simulink model "bh_SM_quad_NO_spin_props"  (R2017a)
settings: Solver=ode23t  StartTime=0.0  StopTime=200  FixedStep=0.001  RelTol=1e-5  EnableMultiTasking=on
undefined symbols (not defined in the file): P_elec, P_mot, P_one_prop, P_rot, P_veh, P_veh_no_props, sigbuilder_block, X, xme_dot_0, Y, Z
libraries: bh_6dof_LIBRARY x22, sm_lib x22, nesl_utility x19, simulink_extras x17, simulink x15
(part 2 of 3)

== system bh_SM_quad_NO_spin_props/CONT_SYS Force_Moment_CMDS/PITCH_and_ROLL_CONT/plots ==
  In1 : Inport
  Demux : Demux  Outputs=2
  Demux1 : Demux  Outputs=2
  P_and_R_CMDs : Scope  NumInputPorts=6
  Radians to Degrees : simulink_extras/Transformations/Radians to Degrees
  Radians to Degrees1 : simulink_extras/Transformations/Radians to Degrees
  Radians to Degrees2 : simulink_extras/Transformations/Radians to Degrees
  wires:
  In1/1 -> Demux1/1, Radians to Degrees/1, Demux/1, P_and_R_CMDs/1
  Demux/1 -> P_and_R_CMDs/2  "Pitch_rad"
  Demux/2 -> P_and_R_CMDs/3  "Roll_rad"
  Radians to Degrees/1 -> P_and_R_CMDs/4  "p_and_r_DEG"
  Demux1/1 -> Radians to Degrees2/1
  Demux1/2 -> Radians to Degrees1/1
  Radians to Degrees2/1 -> P_and_R_CMDs/5  "Pitch_DEG"
  Radians to Degrees1/1 -> P_and_R_CMDs/6  "Roll_DEG"

== system bh_SM_quad_NO_spin_props/CONT_SYS Force_Moment_CMDS/PITCH_and_ROLL_CONT/psi ==
  In1 : Inport
  Bus Selector1 : BusSelector  OutputSignals=phi_theta_psi
  Bus Selector2 : BusSelector  OutputSignals=DOT_phi_theta_psi
  Selector1 : Selector  InputPortWidth=3  IndexOptions=Index vector (dialog)  Indices=3  OutputSizes=1
  Selector2 : Selector  InputPortWidth=3  IndexOptions=Index vector (dialog)  Indices=3  OutputSizes=1
  Out1 : Outport
  Out2 : Outport  Port=2
  wires:
  In1/1 -> Bus Selector2/1, Bus Selector1/1
  Selector1/1 -> Out1/1
  Bus Selector1/1 -> Selector1/1  "<phi_theta_psi>"
  Bus Selector2/1 -> Selector2/1  "<DOT_phi_theta_psi>"
  Selector2/1 -> Out2/1

== system bh_SM_quad_NO_spin_props/CONT_SYS Force_Moment_CMDS/PITCH_and_ROLL_CONT/theta ==
  In1 : Inport
  Bus Selector1 : BusSelector  OutputSignals=phi_theta_psi
  Bus Selector2 : BusSelector  OutputSignals=DOT_phi_theta_psi
  Selector1 : Selector  InputPortWidth=3  IndexOptions=Index vector (dialog)  Indices=2  OutputSizes=1
  Selector2 : Selector  InputPortWidth=3  IndexOptions=Index vector (dialog)  Indices=2  OutputSizes=1
  Out1 : Outport
  Out2 : Outport  Port=2
  wires:
  In1/1 -> Bus Selector2/1, Bus Selector1/1
  Selector1/1 -> Out1/1
  Bus Selector1/1 -> Selector1/1  "<phi_theta_psi>"
  Bus Selector2/1 -> Selector2/1  "<DOT_phi_theta_psi>"
  Selector2/1 -> Out2/1

== system bh_SM_quad_NO_spin_props/CONT_SYS Force_Moment_CMDS/YAW_CONT/FINAL_DES_YAW_CONTROL_SYSTEM ==
  note: NOTE: 1 radian = 57 degrees
  YAW_CMD : Inport
  YAW_MEAS : Inport  Port=2
  YAW_dot_MEAS : Inport  Port=3
  P_CONT_too : simulink/Continuous/PID Controller  Controller=P  TimeDomain=Continuous-time  SampleTime=-1  IntegratorMethod=Forward Euler  FilterMethod=Forward Euler  Form=Parallel  UseFilter=on  ControllerParametersSource=internal  P=1.61636567778084  I=0.151389824684851  D=0  N=100  InitialConditionSource=internal  InitialConditionForIntegrator=0  InitialConditionForFilter=0  ExternalReset=none  LimitOutput=off  UpperSaturationLimit=inf  LowerSaturationLimit=-inf  LinearizeAsGain=on  AntiWindupMode=none  Kb=1  TrackingMode=off  Kt=1  PParamMin=[]  PParamMax=[]  IParamMin=[]  IParamMax=[]  DParamMin=[]  DParamMax=[]  NParamMin=[]  NParamMax=[]  KbParamMin=[]  KbParamMax=[]  KtParamMin=[]  KtParamMax=[]  POutMin=[]  POutMax=[]  IOutMin=[]  IOutMax=[]  DOutMin=[]  DOutMax=[]  NOutMin=[]  NOutMax=[]  KbOutMin=[]  KbOutMax=[]  KtOutMin=[]  KtOutMax=[]  IntegratorOutMin=[]  IntegratorOutMax=[]  FilterOutMin=[]  FilterOutMax=[]  SumOutMin=[]  SumOutMax=[]  SumI1OutMin=[]  SumI1OutMax=[]  SumI2OutMin=[]  SumI2OutMax=[]  SumI3OutMin=[]  SumI3OutMax=[]  SumDOutMin=[]  SumDOutMax=[]  SaturationOutMin=[]  SaturationOutMax=[]  IntegratorContinuousStateAttributes=''  IntegratorStateMustResolveToSignalObject=off  IntegratorRTWStateStorageClass=Auto  FilterContinuousStateAttributes=''  FilterStateMustResolveToSignalObject=off  FilterRTWStateStorageClass=Auto  DifferentiatorICPrevScaledInput=0  DifferentiatorOutMin=[]  DifferentiatorOutMax=[]  InitialConditionSetting=State (most efficient)
  P_Cont : simulink/Continuous/PID Controller  Controller=P  TimeDomain=Continuous-time  SampleTime=-1  IntegratorMethod=Forward Euler  FilterMethod=Forward Euler  Form=Parallel  UseFilter=on  ControllerParametersSource=internal  P=0.09744859506471  I=7.09690484808648  D=-0.334898279224841  N=17.076664592689  InitialConditionSource=internal  InitialConditionForIntegrator=0  InitialConditionForFilter=0  ExternalReset=none  LimitOutput=off  UpperSaturationLimit=inf  LowerSaturationLimit=-inf  LinearizeAsGain=on  AntiWindupMode=none  Kb=1  TrackingMode=off  Kt=1  PParamMin=[]  PParamMax=[]  IParamMin=[]  IParamMax=[]  DParamMin=[]  DParamMax=[]  NParamMin=[]  NParamMax=[]  KbParamMin=[]  KbParamMax=[]  KtParamMin=[]  KtParamMax=[]  POutMin=[]  POutMax=[]  IOutMin=[]  IOutMax=[]  DOutMin=[]  DOutMax=[]  NOutMin=[]  NOutMax=[]  KbOutMin=[]  KbOutMax=[]  KtOutMin=[]  KtOutMax=[]  IntegratorOutMin=[]  IntegratorOutMax=[]  FilterOutMin=[]  FilterOutMax=[]  SumOutMin=[]  SumOutMax=[]  SumI1OutMin=[]  SumI1OutMax=[]  SumI2OutMin=[]  SumI2OutMax=[]  SumI3OutMin=[]  SumI3OutMax=[]  SumDOutMin=[]  SumDOutMax=[]  SaturationOutMin=[]  SaturationOutMax=[]  IntegratorContinuousStateAttributes=''  IntegratorStateMustResolveToSignalObject=off  IntegratorRTWStateStorageClass=Auto  FilterContinuousStateAttributes=''  FilterStateMustResolveToSignalObject=off  FilterRTWStateStorageClass=Auto  DifferentiatorICPrevScaledInput=0  DifferentiatorOutMin=[]  DifferentiatorOutMax=[]  InitialConditionSetting=State (most efficient)
  Sum1 : Sum  Inputs=|+-
  Sum3 : Sum  Inputs=|+-
  TQ_YAW : Outport
  wires:
  Sum3/1 -> P_Cont/1
  P_Cont/1 -> TQ_YAW/1  "TQ"
  YAW_CMD/1 -> Sum1/1
  YAW_MEAS/1 -> Sum1/2
  YAW_dot_MEAS/1 -> Sum3/2
  Sum1/1 -> P_CONT_too/1
  P_CONT_too/1 -> Sum3/1

== system bh_SM_quad_NO_spin_props/CONT_SYS Force_Moment_CMDS/Z_CONT/FINAL_DES_ALTITUDE_CONTROL_SYSTEM ==
  Ze_CMD : Inport
  Ze_MEAS : Inport  Port=2
  Ze_dot_MEAS : Inport  Port=3
  P_cont : simulink/Continuous/PID Controller  Controller=P  TimeDomain=Continuous-time  SampleTime=-1  IntegratorMethod=Forward Euler  FilterMethod=Forward Euler  Form=Parallel  UseFilter=on  ControllerParametersSource=internal  P=6.7862699178667  I=7.09690484808648  D=-0.334898279224841  N=17.076664592689  InitialConditionSource=internal  InitialConditionForIntegrator=0  InitialConditionForFilter=0  ExternalReset=none  LimitOutput=off  UpperSaturationLimit=inf  LowerSaturationLimit=-inf  LinearizeAsGain=on  AntiWindupMode=none  Kb=1  TrackingMode=off  Kt=1  PParamMin=[]  PParamMax=[]  IParamMin=[]  IParamMax=[]  DParamMin=[]  DParamMax=[]  NParamMin=[]  NParamMax=[]  KbParamMin=[]  KbParamMax=[]  KtParamMin=[]  KtParamMax=[]  POutMin=[]  POutMax=[]  IOutMin=[]  IOutMax=[]  DOutMin=[]  DOutMax=[]  NOutMin=[]  NOutMax=[]  KbOutMin=[]  KbOutMax=[]  KtOutMin=[]  KtOutMax=[]  IntegratorOutMin=[]  IntegratorOutMax=[]  FilterOutMin=[]  FilterOutMax=[]  SumOutMin=[]  SumOutMax=[]  SumI1OutMin=[]  SumI1OutMax=[]  SumI2OutMin=[]  SumI2OutMax=[]  SumI3OutMin=[]  SumI3OutMax=[]  SumDOutMin=[]  SumDOutMax=[]  SaturationOutMin=[]  SaturationOutMax=[]  IntegratorContinuousStateAttributes=''  IntegratorStateMustResolveToSignalObject=off  IntegratorRTWStateStorageClass=Auto  FilterContinuousStateAttributes=''  FilterStateMustResolveToSignalObject=off  FilterRTWStateStorageClass=Auto  DifferentiatorICPrevScaledInput=0  DifferentiatorOutMin=[]  DifferentiatorOutMax=[]  InitialConditionSetting=State (most efficient)
  P_cont_too : simulink/Continuous/PID Controller  Controller=P  TimeDomain=Continuous-time  SampleTime=-1  IntegratorMethod=Forward Euler  FilterMethod=Forward Euler  Form=Parallel  UseFilter=on  ControllerParametersSource=internal  P=0.931782439164433  I=0.151389824684851  D=0.117353405685993  N=2.94633103429336  InitialConditionSource=internal  InitialConditionForIntegrator=0  InitialConditionForFilter=0  ExternalReset=none  LimitOutput=off  UpperSaturationLimit=inf  LowerSaturationLimit=-inf  LinearizeAsGain=on  AntiWindupMode=none  Kb=1  TrackingMode=off  Kt=1  PParamMin=[]  PParamMax=[]  IParamMin=[]  IParamMax=[]  DParamMin=[]  DParamMax=[]  NParamMin=[]  NParamMax=[]  KbParamMin=[]  KbParamMax=[]  KtParamMin=[]  KtParamMax=[]  POutMin=[]  POutMax=[]  IOutMin=[]  IOutMax=[]  DOutMin=[]  DOutMax=[]  NOutMin=[]  NOutMax=[]  KbOutMin=[]  KbOutMax=[]  KtOutMin=[]  KtOutMax=[]  IntegratorOutMin=[]  IntegratorOutMax=[]  FilterOutMin=[]  FilterOutMax=[]  SumOutMin=[]  SumOutMax=[]  SumI1OutMin=[]  SumI1OutMax=[]  SumI2OutMin=[]  SumI2OutMax=[]  SumI3OutMin=[]  SumI3OutMax=[]  SumDOutMin=[]  SumDOutMax=[]  SaturationOutMin=[]  SaturationOutMax=[]  IntegratorContinuousStateAttributes=''  IntegratorStateMustResolveToSignalObject=off  IntegratorRTWStateStorageClass=Auto  FilterContinuousStateAttributes=''  FilterStateMustResolveToSignalObject=off  FilterRTWStateStorageClass=Auto  DifferentiatorICPrevScaledInput=0  DifferentiatorOutMin=[]  DifferentiatorOutMax=[]  InitialConditionSetting=State (most efficient)
  Sum1 : Sum  Inputs=|+-
  Sum3 : Sum  Inputs=|+-
  THRUST : Outport
  wires:
  Sum1/1 -> P_cont_too/1
  Sum3/1 -> P_cont/1
  Ze_CMD/1 -> Sum1/1
  P_cont/1 -> THRUST/1  "THRUST"
  P_cont_too/1 -> Sum3/1
  Ze_MEAS/1 -> Sum1/2
  Ze_dot_MEAS/1 -> Sum3/2

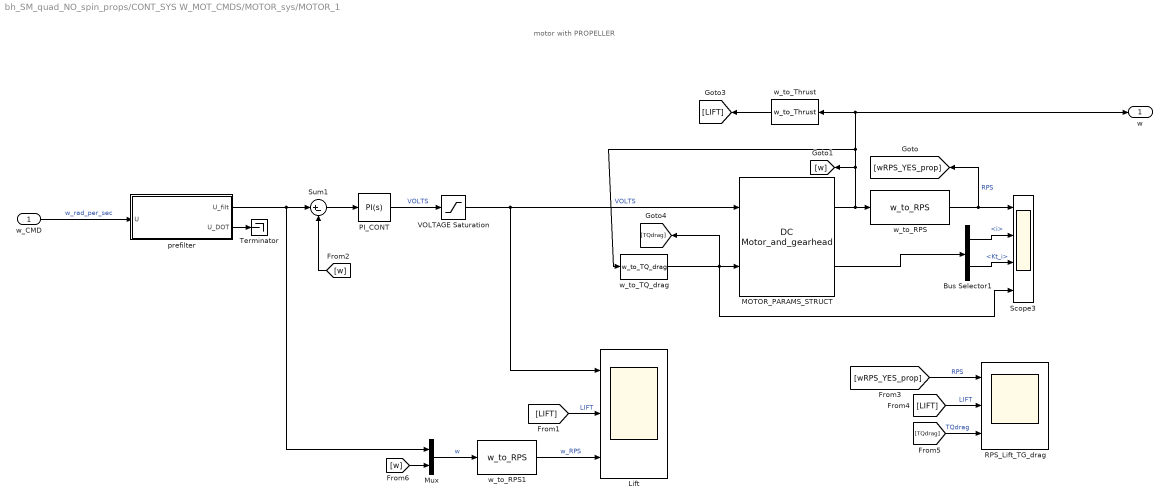
== system bh_SM_quad_NO_spin_props/CONT_SYS W_MOT_CMDS/MOTOR_sys/MOTOR_1 ==
  note: motor with PROPELLER
  w_CMD : Inport
  Bus Selector1 : BusSelector  OutputSignals=Elec.i,TQ_mot.Kt_i
  Lift : Scope  NumInputPorts=3
  MOTOR_PARAMS_STRUCT : bh_6dof_LIBRARY/MODELS/DC Motor_and_gearhead  K=P_mot.Ka  B=P_mot.b  J=P_mot.I  R=P_mot.R  L=P_mot.L  Kb=P_mot.Ke  ID=P_mot.ID
  Mux : Mux  Inputs=2
  PI_CONT : simulink/Continuous/PID Controller  Controller=PI  TimeDomain=Continuous-time  SampleTime=-1  IntegratorMethod=Forward Euler  FilterMethod=Forward Euler  Form=Parallel  UseFilter=on  ControllerParametersSource=internal  P=2.97678216835849  I=24.9655384194189  D=-0.0417302954853434  N=6.67624174583517  InitialConditionSource=internal  InitialConditionForIntegrator=0  InitialConditionForFilter=0  ExternalReset=none  LimitOutput=off  UpperSaturationLimit=inf  LowerSaturationLimit=-inf  LinearizeAsGain=on  AntiWindupMode=none  Kb=1  TrackingMode=off  Kt=1  PParamMin=[]  PParamMax=[]  IParamMin=[]  IParamMax=[]  DParamMin=[]  DParamMax=[]  NParamMin=[]  NParamMax=[]  KbParamMin=[]  KbParamMax=[]  KtParamMin=[]  KtParamMax=[]  POutMin=[]  POutMax=[]  IOutMin=[]  IOutMax=[]  DOutMin=[]  DOutMax=[]  NOutMin=[]  NOutMax=[]  KbOutMin=[]  KbOutMax=[]  KtOutMin=[]  KtOutMax=[]  IntegratorOutMin=[]  IntegratorOutMax=[]  FilterOutMin=[]  FilterOutMax=[]  SumOutMin=[]  SumOutMax=[]  SumI1OutMin=[]  SumI1OutMax=[]  SumI2OutMin=[]  SumI2OutMax=[]  SumI3OutMin=[]  SumI3OutMax=[]  SumDOutMin=[]  SumDOutMax=[]  SaturationOutMin=[]  SaturationOutMax=[]  IntegratorContinuousStateAttributes=''  IntegratorStateMustResolveToSignalObject=off  IntegratorRTWStateStorageClass=Auto  FilterContinuousStateAttributes=''  FilterStateMustResolveToSignalObject=off  FilterRTWStateStorageClass=Auto  DifferentiatorICPrevScaledInput=0  DifferentiatorOutMin=[]  DifferentiatorOutMax=[]  InitialConditionSetting=State (most efficient)
  RPS_Lift_TG_drag : Scope  NumInputPorts=3
  Scope3 : Scope  NumInputPorts=4
  Sum1 : Sum  Inputs=|+-
  Terminator : Terminator
  VOLTAGE Saturation : Saturate  UpperLimit=P_elec.V_mot_max  LowerLimit=P_elec.V_mot_min
      settings: AttributesFormatString=|
      | Vmax = %<UpperLimit>
      | Vmin = %<LowerLimit>
  prefilter : Subsystem  mask(Derivative Estimation){wn=2*pi*5, p=1}
      mask prompts: wn "Natural frequency, wn (rad/sec)"; p "Damping ratio, p"
      mask help:
      | A simple derivative estimator using a 2nd order representation between input and output.
      |
      | The integrators use a discrete FORWARd Euler rule, and a sample time needs to be specified.
      mask init:
      | str1 = sprintf('wn = %.2f', wn);
      | str2 = sprintf('p  = %.2f', p);
      | %str3 = sprintf('dt = %.2f', dt);
      | %str = char(str1,str2,str3);
      | %str3 = sprintf('dt = %.2f', dt);
      | str = char(str1,str2);
      mask Display: disp(str)
  w_to_RPS : bh_6dof_LIBRARY/MODELS/w_to_RPS  SystemSampleTime=-1
  w_to_RPS1 : bh_6dof_LIBRARY/MODELS/w_to_RPS  SystemSampleTime=-1
  w_to_TQ_drag : bh_6dof_LIBRARY/MODELS/w_to_TQ_drag  k=P_one_prop.TWIST_per_w2
  w_to_Thrust : bh_6dof_LIBRARY/MODELS/w_to_Thrust  k=P_one_prop.LIFT_per_w2
  w : Outport
  wires:
  VOLTAGE Saturation/1 -> Lift/1, MOTOR_PARAMS_STRUCT/1  "VOLTS"
  [TQdrag] -> RPS_Lift_TG_drag/3  "TQdrag"
  Sum1/1 -> PI_CONT/1
  w_to_TQ_drag/1 -> [TQdrag], MOTOR_PARAMS_STRUCT/2, Scope3/4
  [LIFT] -> RPS_Lift_TG_drag/2  "LIFT"
  [wRPS_YES_prop] -> RPS_Lift_TG_drag/1  "RPS"
  w_to_Thrust/1 -> [LIFT]
  w_to_RPS/1 -> [wRPS_YES_prop], Scope3/1  "RPS"
  Bus Selector1/1 -> Scope3/2  "<i>"
  MOTOR_PARAMS_STRUCT/2 -> Bus Selector1/1
  Bus Selector1/2 -> Scope3/3  "<Kt_i>"
  MOTOR_PARAMS_STRUCT/1 -> w_to_RPS/1, [w], w/1, w_to_Thrust/1, w_to_TQ_drag/1
  [w] -> Sum1/2
  [LIFT] -> Lift/2  "LIFT"
  Mux/1 -> w_to_RPS1/1  "w"
  [w] -> Mux/2
  w_to_RPS1/1 -> Lift/3  "w_RPS"
  PI_CONT/1 -> VOLTAGE Saturation/1  "VOLTS"
  w_CMD/1 -> prefilter/1(U)  "w_rad_per_sec"
  prefilter/1(U_filt) -> Mux/1, Sum1/1
  prefilter/2(U_DOT) -> Terminator/1

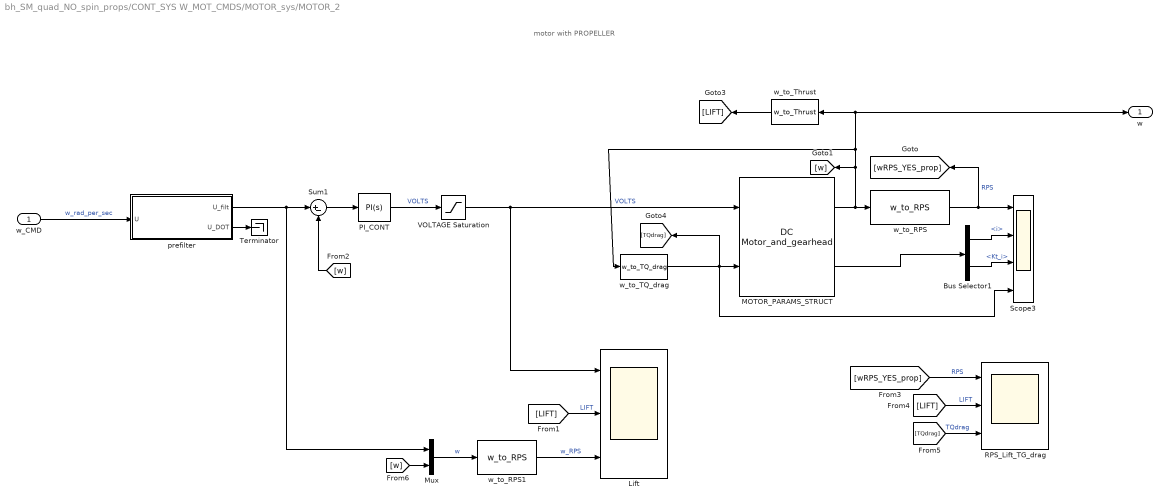
== system bh_SM_quad_NO_spin_props/CONT_SYS W_MOT_CMDS/MOTOR_sys/MOTOR_2 ==
  note: motor with PROPELLER
  w_CMD : Inport
  Bus Selector1 : BusSelector  OutputSignals=Elec.i,TQ_mot.Kt_i
  Lift : Scope  NumInputPorts=3
  MOTOR_PARAMS_STRUCT : bh_6dof_LIBRARY/MODELS/DC Motor_and_gearhead  K=P_mot.Ka  B=P_mot.b  J=P_mot.I  R=P_mot.R  L=P_mot.L  Kb=P_mot.Ke  ID=P_mot.ID
  Mux : Mux  Inputs=2
  PI_CONT : simulink/Continuous/PID Controller  Controller=PI  TimeDomain=Continuous-time  SampleTime=-1  IntegratorMethod=Forward Euler  FilterMethod=Forward Euler  Form=Parallel  UseFilter=on  ControllerParametersSource=internal  P=2.97678216835849  I=24.9655384194189  D=-0.0417302954853434  N=6.67624174583517  InitialConditionSource=internal  InitialConditionForIntegrator=0  InitialConditionForFilter=0  ExternalReset=none  LimitOutput=off  UpperSaturationLimit=inf  LowerSaturationLimit=-inf  LinearizeAsGain=on  AntiWindupMode=none  Kb=1  TrackingMode=off  Kt=1  PParamMin=[]  PParamMax=[]  IParamMin=[]  IParamMax=[]  DParamMin=[]  DParamMax=[]  NParamMin=[]  NParamMax=[]  KbParamMin=[]  KbParamMax=[]  KtParamMin=[]  KtParamMax=[]  POutMin=[]  POutMax=[]  IOutMin=[]  IOutMax=[]  DOutMin=[]  DOutMax=[]  NOutMin=[]  NOutMax=[]  KbOutMin=[]  KbOutMax=[]  KtOutMin=[]  KtOutMax=[]  IntegratorOutMin=[]  IntegratorOutMax=[]  FilterOutMin=[]  FilterOutMax=[]  SumOutMin=[]  SumOutMax=[]  SumI1OutMin=[]  SumI1OutMax=[]  SumI2OutMin=[]  SumI2OutMax=[]  SumI3OutMin=[]  SumI3OutMax=[]  SumDOutMin=[]  SumDOutMax=[]  SaturationOutMin=[]  SaturationOutMax=[]  IntegratorContinuousStateAttributes=''  IntegratorStateMustResolveToSignalObject=off  IntegratorRTWStateStorageClass=Auto  FilterContinuousStateAttributes=''  FilterStateMustResolveToSignalObject=off  FilterRTWStateStorageClass=Auto  DifferentiatorICPrevScaledInput=0  DifferentiatorOutMin=[]  DifferentiatorOutMax=[]  InitialConditionSetting=State (most efficient)
  RPS_Lift_TG_drag : Scope  NumInputPorts=3
  Scope3 : Scope  NumInputPorts=4
  Sum1 : Sum  Inputs=|+-
  Terminator : Terminator
  VOLTAGE Saturation : Saturate  UpperLimit=P_elec.V_mot_max  LowerLimit=P_elec.V_mot_min
      settings: AttributesFormatString=|
      | Vmax = %<UpperLimit>
      | Vmin = %<LowerLimit>
  prefilter : Subsystem  mask(Derivative Estimation){wn=2*pi*5, p=1}
      mask prompts: wn "Natural frequency, wn (rad/sec)"; p "Damping ratio, p"
      mask help:
      | A simple derivative estimator using a 2nd order representation between input and output.
      |
      | The integrators use a discrete FORWARd Euler rule, and a sample time needs to be specified.
      mask init:
      | str1 = sprintf('wn = %.2f', wn);
      | str2 = sprintf('p  = %.2f', p);
      | %str3 = sprintf('dt = %.2f', dt);
      | %str = char(str1,str2,str3);
      | %str3 = sprintf('dt = %.2f', dt);
      | str = char(str1,str2);
      mask Display: disp(str)
  w_to_RPS : bh_6dof_LIBRARY/MODELS/w_to_RPS  SystemSampleTime=-1
  w_to_RPS1 : bh_6dof_LIBRARY/MODELS/w_to_RPS  SystemSampleTime=-1
  w_to_TQ_drag : bh_6dof_LIBRARY/MODELS/w_to_TQ_drag  k=P_one_prop.TWIST_per_w2
  w_to_Thrust : bh_6dof_LIBRARY/MODELS/w_to_Thrust  k=P_one_prop.LIFT_per_w2
  w : Outport
  wires:
  VOLTAGE Saturation/1 -> Lift/1, MOTOR_PARAMS_STRUCT/1  "VOLTS"
  [TQdrag] -> RPS_Lift_TG_drag/3  "TQdrag"
  Sum1/1 -> PI_CONT/1
  w_to_TQ_drag/1 -> [TQdrag], MOTOR_PARAMS_STRUCT/2, Scope3/4
  [LIFT] -> RPS_Lift_TG_drag/2  "LIFT"
  [wRPS_YES_prop] -> RPS_Lift_TG_drag/1  "RPS"
  w_to_Thrust/1 -> [LIFT]
  w_to_RPS/1 -> [wRPS_YES_prop], Scope3/1  "RPS"
  Bus Selector1/1 -> Scope3/2  "<i>"
  MOTOR_PARAMS_STRUCT/2 -> Bus Selector1/1
  Bus Selector1/2 -> Scope3/3  "<Kt_i>"
  MOTOR_PARAMS_STRUCT/1 -> w_to_RPS/1, [w], w/1, w_to_Thrust/1, w_to_TQ_drag/1
  [w] -> Sum1/2
  [LIFT] -> Lift/2  "LIFT"
  Mux/1 -> w_to_RPS1/1  "w"
  [w] -> Mux/2
  w_to_RPS1/1 -> Lift/3  "w_RPS"
  PI_CONT/1 -> VOLTAGE Saturation/1  "VOLTS"
  w_CMD/1 -> prefilter/1(U)  "w_rad_per_sec"
  prefilter/1(U_filt) -> Mux/1, Sum1/1
  prefilter/2(U_DOT) -> Terminator/1

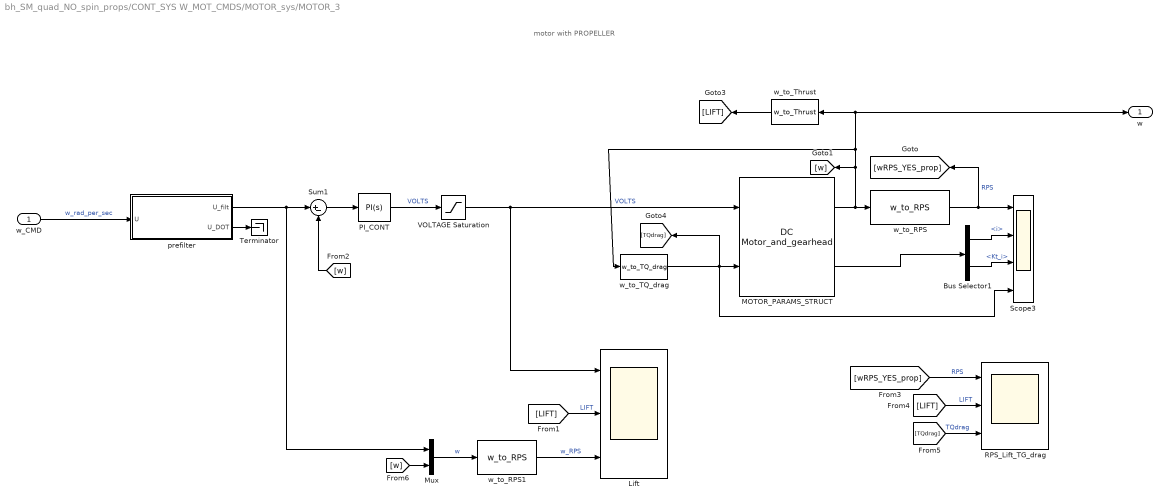
== system bh_SM_quad_NO_spin_props/CONT_SYS W_MOT_CMDS/MOTOR_sys/MOTOR_3 ==
  note: motor with PROPELLER
  w_CMD : Inport
  Bus Selector1 : BusSelector  OutputSignals=Elec.i,TQ_mot.Kt_i
  Lift : Scope  NumInputPorts=3
  MOTOR_PARAMS_STRUCT : bh_6dof_LIBRARY/MODELS/DC Motor_and_gearhead  K=P_mot.Ka  B=P_mot.b  J=P_mot.I  R=P_mot.R  L=P_mot.L  Kb=P_mot.Ke  ID=P_mot.ID
  Mux : Mux  Inputs=2
  PI_CONT : simulink/Continuous/PID Controller  Controller=PI  TimeDomain=Continuous-time  SampleTime=-1  IntegratorMethod=Forward Euler  FilterMethod=Forward Euler  Form=Parallel  UseFilter=on  ControllerParametersSource=internal  P=2.97678216835849  I=24.9655384194189  D=-0.0417302954853434  N=6.67624174583517  InitialConditionSource=internal  InitialConditionForIntegrator=0  InitialConditionForFilter=0  ExternalReset=none  LimitOutput=off  UpperSaturationLimit=inf  LowerSaturationLimit=-inf  LinearizeAsGain=on  AntiWindupMode=none  Kb=1  TrackingMode=off  Kt=1  PParamMin=[]  PParamMax=[]  IParamMin=[]  IParamMax=[]  DParamMin=[]  DParamMax=[]  NParamMin=[]  NParamMax=[]  KbParamMin=[]  KbParamMax=[]  KtParamMin=[]  KtParamMax=[]  POutMin=[]  POutMax=[]  IOutMin=[]  IOutMax=[]  DOutMin=[]  DOutMax=[]  NOutMin=[]  NOutMax=[]  KbOutMin=[]  KbOutMax=[]  KtOutMin=[]  KtOutMax=[]  IntegratorOutMin=[]  IntegratorOutMax=[]  FilterOutMin=[]  FilterOutMax=[]  SumOutMin=[]  SumOutMax=[]  SumI1OutMin=[]  SumI1OutMax=[]  SumI2OutMin=[]  SumI2OutMax=[]  SumI3OutMin=[]  SumI3OutMax=[]  SumDOutMin=[]  SumDOutMax=[]  SaturationOutMin=[]  SaturationOutMax=[]  IntegratorContinuousStateAttributes=''  IntegratorStateMustResolveToSignalObject=off  IntegratorRTWStateStorageClass=Auto  FilterContinuousStateAttributes=''  FilterStateMustResolveToSignalObject=off  FilterRTWStateStorageClass=Auto  DifferentiatorICPrevScaledInput=0  DifferentiatorOutMin=[]  DifferentiatorOutMax=[]  InitialConditionSetting=State (most efficient)
  RPS_Lift_TG_drag : Scope  NumInputPorts=3
  Scope3 : Scope  NumInputPorts=4
  Sum1 : Sum  Inputs=|+-
  Terminator : Terminator
  VOLTAGE Saturation : Saturate  UpperLimit=P_elec.V_mot_max  LowerLimit=P_elec.V_mot_min
      settings: AttributesFormatString=|
      | Vmax = %<UpperLimit>
      | Vmin = %<LowerLimit>
  prefilter : Subsystem  mask(Derivative Estimation){wn=2*pi*5, p=1}
      mask prompts: wn "Natural frequency, wn (rad/sec)"; p "Damping ratio, p"
      mask help:
      | A simple derivative estimator using a 2nd order representation between input and output.
      |
      | The integrators use a discrete FORWARd Euler rule, and a sample time needs to be specified.
      mask init:
      | str1 = sprintf('wn = %.2f', wn);
      | str2 = sprintf('p  = %.2f', p);
      | %str3 = sprintf('dt = %.2f', dt);
      | %str = char(str1,str2,str3);
      | %str3 = sprintf('dt = %.2f', dt);
      | str = char(str1,str2);
      mask Display: disp(str)
  w_to_RPS : bh_6dof_LIBRARY/MODELS/w_to_RPS  SystemSampleTime=-1
  w_to_RPS1 : bh_6dof_LIBRARY/MODELS/w_to_RPS  SystemSampleTime=-1
  w_to_TQ_drag : bh_6dof_LIBRARY/MODELS/w_to_TQ_drag  k=P_one_prop.TWIST_per_w2
  w_to_Thrust : bh_6dof_LIBRARY/MODELS/w_to_Thrust  k=P_one_prop.LIFT_per_w2
  w : Outport
  wires:
  VOLTAGE Saturation/1 -> Lift/1, MOTOR_PARAMS_STRUCT/1  "VOLTS"
  [TQdrag] -> RPS_Lift_TG_drag/3  "TQdrag"
  Sum1/1 -> PI_CONT/1
  w_to_TQ_drag/1 -> [TQdrag], MOTOR_PARAMS_STRUCT/2, Scope3/4
  [LIFT] -> RPS_Lift_TG_drag/2  "LIFT"
  [wRPS_YES_prop] -> RPS_Lift_TG_drag/1  "RPS"
  w_to_Thrust/1 -> [LIFT]
  w_to_RPS/1 -> [wRPS_YES_prop], Scope3/1  "RPS"
  Bus Selector1/1 -> Scope3/2  "<i>"
  MOTOR_PARAMS_STRUCT/2 -> Bus Selector1/1
  Bus Selector1/2 -> Scope3/3  "<Kt_i>"
  MOTOR_PARAMS_STRUCT/1 -> w_to_RPS/1, [w], w/1, w_to_Thrust/1, w_to_TQ_drag/1
  [w] -> Sum1/2
  [LIFT] -> Lift/2  "LIFT"
  Mux/1 -> w_to_RPS1/1  "w"
  [w] -> Mux/2
  w_to_RPS1/1 -> Lift/3  "w_RPS"
  PI_CONT/1 -> VOLTAGE Saturation/1  "VOLTS"
  w_CMD/1 -> prefilter/1(U)  "w_rad_per_sec"
  prefilter/1(U_filt) -> Mux/1, Sum1/1
  prefilter/2(U_DOT) -> Terminator/1

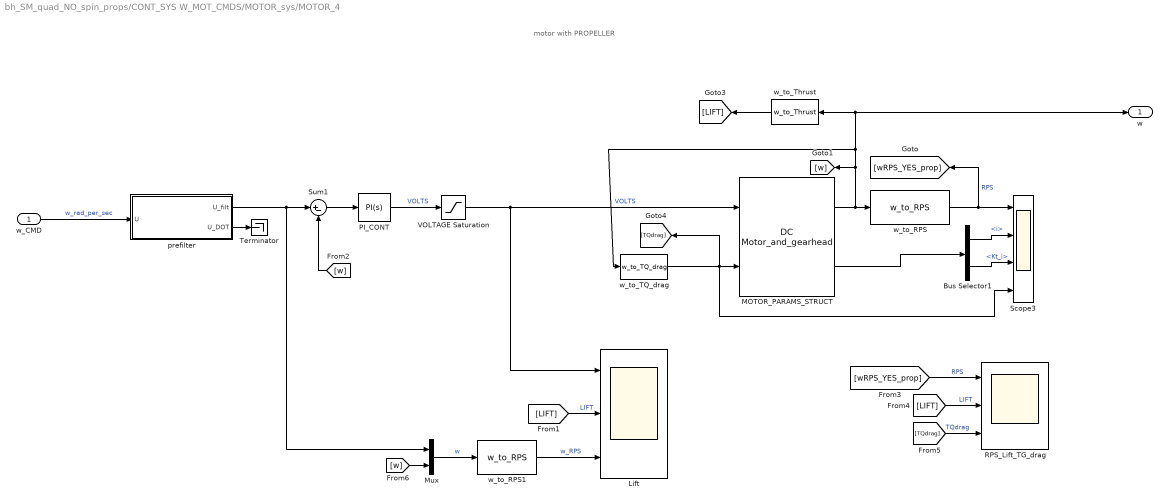
== system bh_SM_quad_NO_spin_props/CONT_SYS W_MOT_CMDS/MOTOR_sys/MOTOR_4 ==
  note: motor with PROPELLER
  w_CMD : Inport
  Bus Selector1 : BusSelector  OutputSignals=Elec.i,TQ_mot.Kt_i
  Lift : Scope  NumInputPorts=3
  MOTOR_PARAMS_STRUCT : bh_6dof_LIBRARY/MODELS/DC Motor_and_gearhead  K=P_mot.Ka  B=P_mot.b  J=P_mot.I  R=P_mot.R  L=P_mot.L  Kb=P_mot.Ke  ID=P_mot.ID
  Mux : Mux  Inputs=2
  PI_CONT : simulink/Continuous/PID Controller  Controller=PI  TimeDomain=Continuous-time  SampleTime=-1  IntegratorMethod=Forward Euler  FilterMethod=Forward Euler  Form=Parallel  UseFilter=on  ControllerParametersSource=internal  P=2.97678216835849  I=24.9655384194189  D=-0.0417302954853434  N=6.67624174583517  InitialConditionSource=internal  InitialConditionForIntegrator=0  InitialConditionForFilter=0  ExternalReset=none  LimitOutput=off  UpperSaturationLimit=inf  LowerSaturationLimit=-inf  LinearizeAsGain=on  AntiWindupMode=none  Kb=1  TrackingMode=off  Kt=1  PParamMin=[]  PParamMax=[]  IParamMin=[]  IParamMax=[]  DParamMin=[]  DParamMax=[]  NParamMin=[]  NParamMax=[]  KbParamMin=[]  KbParamMax=[]  KtParamMin=[]  KtParamMax=[]  POutMin=[]  POutMax=[]  IOutMin=[]  IOutMax=[]  DOutMin=[]  DOutMax=[]  NOutMin=[]  NOutMax=[]  KbOutMin=[]  KbOutMax=[]  KtOutMin=[]  KtOutMax=[]  IntegratorOutMin=[]  IntegratorOutMax=[]  FilterOutMin=[]  FilterOutMax=[]  SumOutMin=[]  SumOutMax=[]  SumI1OutMin=[]  SumI1OutMax=[]  SumI2OutMin=[]  SumI2OutMax=[]  SumI3OutMin=[]  SumI3OutMax=[]  SumDOutMin=[]  SumDOutMax=[]  SaturationOutMin=[]  SaturationOutMax=[]  IntegratorContinuousStateAttributes=''  IntegratorStateMustResolveToSignalObject=off  IntegratorRTWStateStorageClass=Auto  FilterContinuousStateAttributes=''  FilterStateMustResolveToSignalObject=off  FilterRTWStateStorageClass=Auto  DifferentiatorICPrevScaledInput=0  DifferentiatorOutMin=[]  DifferentiatorOutMax=[]  InitialConditionSetting=State (most efficient)
  RPS_Lift_TG_drag : Scope  NumInputPorts=3
  Scope3 : Scope  NumInputPorts=4
  Sum1 : Sum  Inputs=|+-
  Terminator : Terminator
  VOLTAGE Saturation : Saturate  UpperLimit=P_elec.V_mot_max  LowerLimit=P_elec.V_mot_min
      settings: AttributesFormatString=|
      | Vmax = %<UpperLimit>
      | Vmin = %<LowerLimit>
  prefilter : Subsystem  mask(Derivative Estimation){wn=2*pi*5, p=1}
      mask prompts: wn "Natural frequency, wn (rad/sec)"; p "Damping ratio, p"
      mask help:
      | A simple derivative estimator using a 2nd order representation between input and output.
      |
      | The integrators use a discrete FORWARd Euler rule, and a sample time needs to be specified.
      mask init:
      | str1 = sprintf('wn = %.2f', wn);
      | str2 = sprintf('p  = %.2f', p);
      | %str3 = sprintf('dt = %.2f', dt);
      | %str = char(str1,str2,str3);
      | %str3 = sprintf('dt = %.2f', dt);
      | str = char(str1,str2);
      mask Display: disp(str)
  w_to_RPS : bh_6dof_LIBRARY/MODELS/w_to_RPS  SystemSampleTime=-1
  w_to_RPS1 : bh_6dof_LIBRARY/MODELS/w_to_RPS  SystemSampleTime=-1
  w_to_TQ_drag : bh_6dof_LIBRARY/MODELS/w_to_TQ_drag  k=P_one_prop.TWIST_per_w2
  w_to_Thrust : bh_6dof_LIBRARY/MODELS/w_to_Thrust  k=P_one_prop.LIFT_per_w2
  w : Outport
  wires:
  VOLTAGE Saturation/1 -> Lift/1, MOTOR_PARAMS_STRUCT/1  "VOLTS"
  [TQdrag] -> RPS_Lift_TG_drag/3  "TQdrag"
  Sum1/1 -> PI_CONT/1
  w_to_TQ_drag/1 -> [TQdrag], MOTOR_PARAMS_STRUCT/2, Scope3/4
  [LIFT] -> RPS_Lift_TG_drag/2  "LIFT"
  [wRPS_YES_prop] -> RPS_Lift_TG_drag/1  "RPS"
  w_to_Thrust/1 -> [LIFT]
  w_to_RPS/1 -> [wRPS_YES_prop], Scope3/1  "RPS"
  Bus Selector1/1 -> Scope3/2  "<i>"
  MOTOR_PARAMS_STRUCT/2 -> Bus Selector1/1
  Bus Selector1/2 -> Scope3/3  "<Kt_i>"
  MOTOR_PARAMS_STRUCT/1 -> w_to_RPS/1, [w], w/1, w_to_Thrust/1, w_to_TQ_drag/1
  [w] -> Sum1/2
  [LIFT] -> Lift/2  "LIFT"
  Mux/1 -> w_to_RPS1/1  "w"
  [w] -> Mux/2
  w_to_RPS1/1 -> Lift/3  "w_RPS"
  PI_CONT/1 -> VOLTAGE Saturation/1  "VOLTS"
  w_CMD/1 -> prefilter/1(U)  "w_rad_per_sec"
  prefilter/1(U_filt) -> Mux/1, Sum1/1
  prefilter/2(U_DOT) -> Terminator/1

== system bh_SM_quad_NO_spin_props/CONT_SYS W_MOT_CMDS/MOTOR_sys/w_MUX ==
  W_CMD : Inport
  W : Inport  Port=2
  Demux1 : Demux
  Demux2 : Demux
  Mux{,1..3} (4 alike) : Mux  Inputs=2
  w1 : Outport
  w2 : Outport  Port=2
  w3 : Outport  Port=3
  w4 : Outport  Port=4
  wires:
  W_CMD/1 -> Demux2/1
  W/1 -> Demux1/1
  Mux/1 -> w1/1
  Mux1/1 -> w2/1
  Mux3/1 -> w4/1
  Mux2/1 -> w3/1
  Demux2/1 -> Mux/1
  Demux2/2 -> Mux1/1
  Demux2/3 -> Mux2/1
  Demux2/4 -> Mux3/1
  Demux1/1 -> Mux/2
  Demux1/2 -> Mux1/2
  Demux1/3 -> Mux2/2
  Demux1/4 -> Mux3/2

== system bh_SM_quad_NO_spin_props/MODEL_SYS/bh_6DOF (Simscape)/6DOF_JOINT_SYS ==
  note: NOTE:  For the 6-DOF block
      | SENSED positions and velocities are resolved into BASE frame components
      | INITIAL(target) positions and velocities are resolved into BASE frame components
  6-DOF Joint : sm_lib/Joints/6-DOF Joint  SenseConstraintForce=off  SenseConstraintForceX=off  SenseConstraintForceY=off  SenseConstraintForceZ=off  SenseConstraintTorque=off  SenseConstraintTorqueX=off  SenseConstraintTorqueY=off  SenseConstraintTorqueZ=off  SenseTotalForce=off  SenseTotalForceX=off  SenseTotalForceY=off  SenseTotalForceZ=off  SenseTotalTorque=off  SenseTotalTorqueX=off  SenseTotalTorqueY=off  SenseTotalTorqueZ=off  CompositeWrenchDir=FollowerOnBase  CompositeWrenchFrame=BaseFrame  PxEquilibriumPosition=0  PxEquilibriumPositionUnits=m  PxSpringStiffness=0  PxSpringStiffnessUnits=N/m  PxDampingCoefficient=0  PxDampingCoefficientUnits=N/(m/s)  PxTorqueActuationMode=NoTorque  PxMotionActuationMode=ComputedMotion  PxSensePosition=on  PxSenseVelocity=on  PxSenseAcceleration=off  PxSenseTorqueForce=off  PxPositionTargetSpecify=on  PxPositionTargetPriority=High  PxPositionTargetValue=xme_0(1)  PxPositionTargetValueUnits=m  PxVelocityTargetSpecify=on  PxVelocityTargetPriority=High  PxVelocityTargetValue=xme_dot_0(1)  PxVelocityTargetValueUnits=m/s  PyEquilibriumPosition=0  PyEquilibriumPositionUnits=m  PySpringStiffness=0  PySpringStiffnessUnits=N/m  PyDampingCoefficient=0  PyDampingCoefficientUnits=N/(m/s)  PyTorqueActuationMode=NoTorque  PyMotionActuationMode=ComputedMotion  PySensePosition=on  PySenseVelocity=on  PySenseAcceleration=off  PySenseTorqueForce=off  PyPositionTargetSpecify=on  PyPositionTargetPriority=High  PyPositionTargetValue=xme_0(2)  PyPositionTargetValueUnits=m  PyVelocityTargetSpecify=on  PyVelocityTargetPriority=High  PyVelocityTargetValue=xme_dot_0(2)  PyVelocityTargetValueUnits=m/s  PzEquilibriumPosition=0  PzEquilibriumPositionUnits=m  PzSpringStiffness=0  PzSpringStiffnessUnits=N/m  PzDampingCoefficient=0  PzDampingCoefficientUnits=N/(m/s)  PzTorqueActuationMode=NoTorque  PzMotionActuationMode=ComputedMotion  PzSensePosition=on  PzSenseVelocity=on  PzSenseAcceleration=off  PzSenseTorqueForce=off  PzPositionTargetSpecify=on  PzPositionTargetPriority=High  PzPositionTargetValue=xme_0(3)  PzPositionTargetValueUnits=m  PzVelocityTargetSpecify=on  PzVelocityTargetPriority=High  PzVelocityTargetValue=xme_dot_0(3)  PzVelocityTargetValueUnits=m/s  SphDefPosRotationMethod=None  SphDefPosRotationAngleUnits=deg  SphDefPosRotationStandardAxis=+Z  SphDefPosRotationAngle=0.0  SphDefPosRotationArbitraryAxis=[0 0 1]  SphDefPosFollAlignAxisA=+X  SphDefPosBaseAlignAxisA=+Y  SphDefPosFollAlignAxisB=+Y  SphDefPosBaseAlignAxisB=+Z  SphDefPosRotationSequenceAxes=FollowerAxes  SphDefPosRotationSequence=XYX  SphDefPosRotationSequenceAngles=[0 0 0]  SphDefPosRotationSequenceAnglesUnits=deg  SphDefPosRotationMatrix=[1 0 0; 0 1 0; 0 0 1]  SphEqPosRotationMethod=None  SphEqPosRotationAngleUnits=deg  SphEqPosRotationStandardAxis=+Z  SphEqPosRotationAngle=0.0  SphEqPosRotationArbitraryAxis=[0 0 1]  SphEqPosFollAlignAxisA=+X  SphEqPosBaseAlignAxisA=+Y  SphEqPosFollAlignAxisB=+Y  SphEqPosBaseAlignAxisB=+Z  SphEqPosRotationSequenceAxes=FollowerAxes  SphEqPosRotationSequence=XYX  SphEqPosRotationSequenceAngles=[0 0 0]  SphEqPosRotationSequenceAnglesUnits=deg  SphEqPosRotationMatrix=[1 0 0; 0 1 0; 0 0 1]  SphSpringStiffness=0  SphSpringStiffnessUnits=N*m/deg  SphDampingCoefficient=0  SphDampingCoefficientUnits=N*m/(deg/s)  SphActuateTorqueX=off  SphActuateTorqueY=off  SphActuateTorqueZ=off  SphActuateTorque=off  SphTorqueActuationMode=NoTorque  SphMotionActuationMode=ComputedMotion  SphActuationFrame=BaseFrame  SphSensePosition=off  SphSenseVelocityX=off  SphSenseVelocityY=off  SphSenseVelocityZ=off  SphSenseVelocity=off  SphSenseAccelerationX=off  SphSenseAccelerationY=off  SphSenseAccelerationZ=off  SphSenseAcceleration=off  SphSenseTorqueX=off  SphSenseTorqueY=off  SphSenseTorqueZ=off  SphSenseTorqueForce=off  SphSensingFrame=BaseFrame  SphPositionTargetRotationMethod=RotationSequence  SphPositionTargetRotationAngleUnits=deg  SphPositionTargetRotationStandardAxis=+Z  SphPositionTargetRotationAngle=0.0  SphPositionTargetRotationArbitraryAxis=[0 0 1]  SphPositionTargetFollAlignAxisA=+X  SphPositionTargetBaseAlignAxisA=+Y  SphPositionTargetFollAlignAxisB=+Y  SphPositionTargetBaseAlignAxisB=+Z  SphPositionTargetRotationSequenceAxes=FollowerAxes  SphPositionTargetRotationSequence=ZYX  SphPositionTargetRotationSequenceAngles=eul_0  SphPositionTargetRotationSequenceAnglesUnits=rad  SphPositionTargetRotationMatrix=[1 0 0; 0 1 0; 0 0 1]  SphPositionTargetSpecify=on  SphPositionTargetPriority=High  SphVelocityTargetValue=eul_dot_0  SphVelocityTargetValueUnits=rad/s  SphVelocityTargetSpecify=on  SphVelocityTargetPriority=High  SphVelocityTargetInFollowerFrame=on
      settings: AttributesFormatString=|
      | %<PxPositionTargetValue> %<PyPositionTargetValue> %<PzPositionTargetValue>
      | %<PxVelocityTargetValue> %<PyVelocityTargetValue> %<PzVelocityTargetValue>
      | %<SphPositionTargetRotationSequenceAngles>
      | %<SphPositionTargetRotationSequence>
      | %<SphVelocityTargetValue>
  Angular_MEAS : Subsystem
  Mux : Mux  Inputs=6
  PS-Simulink Converter : nesl_utility/PS-Simulink Converter  PhysicalDomain=network_engine_domain  SubClassName=ps_output  LeftPortType=input  RightPortType=output  PseudoPeriodic=off  Frequencies=[]  Unit=m  AffineConversion=off
  PS-Simulink Converter1 : nesl_utility/PS-Simulink Converter  PhysicalDomain=network_engine_domain  SubClassName=ps_output  LeftPortType=input  RightPortType=output  PseudoPeriodic=off  Frequencies=[]  Unit=m  AffineConversion=off
  PS-Simulink Converter2 : nesl_utility/PS-Simulink Converter  PhysicalDomain=network_engine_domain  SubClassName=ps_output  LeftPortType=input  RightPortType=output  PseudoPeriodic=off  Frequencies=[]  Unit=m  AffineConversion=off
  PS-Simulink Converter3 : nesl_utility/PS-Simulink Converter  PhysicalDomain=network_engine_domain  SubClassName=ps_output  LeftPortType=input  RightPortType=output  PseudoPeriodic=off  Frequencies=[]  Unit=m/s  AffineConversion=off
  PS-Simulink Converter4 : nesl_utility/PS-Simulink Converter  PhysicalDomain=network_engine_domain  SubClassName=ps_output  LeftPortType=input  RightPortType=output  PseudoPeriodic=off  Frequencies=[]  Unit=m/s  AffineConversion=off
  PS-Simulink Converter5 : nesl_utility/PS-Simulink Converter  PhysicalDomain=network_engine_domain  SubClassName=ps_output  LeftPortType=input  RightPortType=output  PseudoPeriodic=off  Frequencies=[]  Unit=m/s  AffineConversion=off
  Reshape : Reshape  OutputDimensionality=Column vector (2-D)
  Reshape1 : Reshape  OutputDimensionality=Column vector (2-D)
  Selector : Selector  InputPortWidth=6  IndexOptions=Index vector (dialog)  Indices=[1 3 5]  OutputSizes=1
  Selector1 : Selector  InputPortWidth=6  IndexOptions=Index vector (dialog)  Indices=[2 4 6]  OutputSizes=1
  integrate : Subsystem  Commented=on
  B : PMIOPort  Port=1  Side=Left
  F : PMIOPort  Port=2  Side=Right
  wb : Outport
  bRg : Outport  Port=2
  eul : Outport  Port=3
  eul_rates : Outport  Port=4
  Xe : Outport  Port=5
  Ve : Outport  Port=6
  wires:
  PS-Simulink Converter/1 -> Mux/1
  PS-Simulink Converter3/1 -> Mux/2
  PS-Simulink Converter1/1 -> Mux/3
  PS-Simulink Converter4/1 -> Mux/4
  PS-Simulink Converter2/1 -> Mux/5
  PS-Simulink Converter5/1 -> Mux/6
  Mux/1 -> Selector1/1, Selector/1
  Selector1/1 -> Reshape/1
  Selector/1 -> Reshape1/1
  Reshape1/1 -> Xe/1
  Reshape/1 -> Ve/1
  Angular_MEAS/1(wb) -> wb/1
  Angular_MEAS/2(bRg) -> bRg/1
  Angular_MEAS/3(eul) -> eul/1
  Angular_MEAS/4(eul_rates) -> eul_rates/1
  connections:
  PS-Simulink Converter4/LConn1 -- 6-DOF Joint/RConn5
  PS-Simulink Converter2/LConn1 -- 6-DOF Joint/RConn6
  PS-Simulink Converter/LConn1 -- 6-DOF Joint/RConn2
  PS-Simulink Converter3/LConn1 -- 6-DOF Joint/RConn3
  6-DOF Joint/LConn1 -- Angular_MEAS/LConn1 -- B/RConn1
  PS-Simulink Converter5/LConn1 -- 6-DOF Joint/RConn7
  PS-Simulink Converter1/LConn1 -- 6-DOF Joint/RConn4
  6-DOF Joint/RConn1 -- Angular_MEAS/RConn1 -- F/RConn1

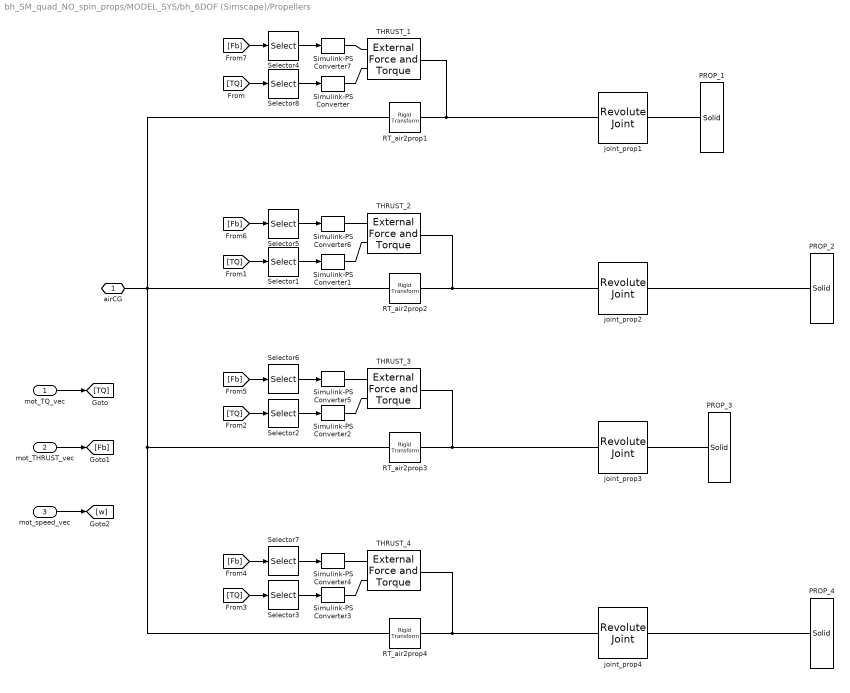
== system bh_SM_quad_NO_spin_props/MODEL_SYS/bh_6DOF (Simscape)/Propellers ==
  mot_TQ_vec : Inport
  mot_THRUST_vec : Inport  Port=2
  mot_speed_vec : Inport  Port=3
  PROP_1 : sm_lib/Body Elements/Solid  InertiaType=Custom  Mass=prop_mass  MassUnits=kg  CenterOfMass=[0 0 0]  CenterOfMassUnits=m  MomentsOfInertia=Iprop_xx_yy_zz  MomentsOfInertiaUnits=kg*m^2  ProductsOfInertia=Iprop_yz_zx_xy  ProductsOfInertiaUnits=kg*m^2  DensityBased=on  Density=1000  DensityUnits=kg/(m^3)  DoExposeReferenceFrame=on  SerializedFrames=<Frames/>  GraphicType=FromGeometry  MarkerShape=Sphere  MarkerSize=10  MarkerSizeUnits=m  GraphicVisPropType=SimpleVisualProperties  GraphicDiffuseColor=[0.0 0.0 1.0]  GraphicSpecularColor=[0.5 0.5 0.5 1.0]  GraphicAmbientColor=[0.15 0.15 0.15 1.0]  GraphicEmissiveColor=[0.0 0.0 0.0 1.0]  GraphicShininess=75  GraphicOpacity=1.0  GeometryShape=Cylinder  RectangleSize=[1 1]  RectangleSizeUnits=m  BrickDimensions=[1 1 1]  BrickDimensionUnits=m  CylinderRadius=prop_CG_H  CylinderRadiusUnits=m  CylinderLength=2*prop_CG_H  CylinderLengthUnits=m  SphereRadius=1  SphereRadiusUnits=m  EllipsoidRadii=[prop_CG_L, prop_CG_L, prop_CG_L/10]  EllipsoidRadiiUnits=m  ExtrusionCrossSection=[1 1; -1 1; -1 -1; 1 -1]  ExtrusionCrossSectionUnits=m  ExtrusionLength=1  ExtrusionLengthUnits=m  PolygonNumSides=3  PolygonOuterRadius=1  PolygonOuterRadiusUnits=m  ExtGeomFileType=STL  ExtGeomFileUnits=m  RevolutionCrossSection=[1 1; 1 -1; 2 -1; 2 1]  RevolutionCrossSectionUnits=m  RevolutionExtent=Full  RevolutionAngle=180  RevolutionAngleUnits=deg
      settings: AttributesFormatString=|
      | %<Mass>
      | %<MomentsOfInertia>
      | %<ProductsOfInertia>
  PROP_2 : sm_lib/Body Elements/Solid  InertiaType=Custom  Mass=prop_mass  MassUnits=kg  CenterOfMass=[0 0 0]  CenterOfMassUnits=m  MomentsOfInertia=Iprop_xx_yy_zz  MomentsOfInertiaUnits=kg*m^2  ProductsOfInertia=Iprop_yz_zx_xy  ProductsOfInertiaUnits=kg*m^2  DensityBased=on  Density=1000  DensityUnits=kg/(m^3)  DoExposeReferenceFrame=on  SerializedFrames=<Frames/>  GraphicType=FromGeometry  MarkerShape=Sphere  MarkerSize=10  MarkerSizeUnits=m  GraphicVisPropType=SimpleVisualProperties  GraphicDiffuseColor=[0.8 0.8 1.0]  GraphicSpecularColor=[0.5 0.5 0.5 1.0]  GraphicAmbientColor=[0.15 0.15 0.15 1.0]  GraphicEmissiveColor=[0.0 0.0 0.0 1.0]  GraphicShininess=75  GraphicOpacity=1.0  GeometryShape=Cylinder  RectangleSize=[1 1]  RectangleSizeUnits=m  BrickDimensions=[1 1 1]  BrickDimensionUnits=m  CylinderRadius=prop_CG_H  CylinderRadiusUnits=m  CylinderLength=2*prop_CG_H  CylinderLengthUnits=m  SphereRadius=1  SphereRadiusUnits=m  EllipsoidRadii=[prop_CG_L, prop_CG_L, prop_CG_L/10]  EllipsoidRadiiUnits=m  ExtrusionCrossSection=[1 1; -1 1; -1 -1; 1 -1]  ExtrusionCrossSectionUnits=m  ExtrusionLength=1  ExtrusionLengthUnits=m  PolygonNumSides=3  PolygonOuterRadius=1  PolygonOuterRadiusUnits=m  ExtGeomFileType=STL  ExtGeomFileUnits=m  RevolutionCrossSection=[1 1; 1 -1; 2 -1; 2 1]  RevolutionCrossSectionUnits=m  RevolutionExtent=Full  RevolutionAngle=180  RevolutionAngleUnits=deg
      settings: AttributesFormatString=|
      | %<Mass>
      | %<MomentsOfInertia>
      | %<ProductsOfInertia>
  PROP_3 : sm_lib/Body Elements/Solid  InertiaType=Custom  Mass=prop_mass  MassUnits=kg  CenterOfMass=[0 0 0]  CenterOfMassUnits=m  MomentsOfInertia=Iprop_xx_yy_zz  MomentsOfInertiaUnits=kg*m^2  ProductsOfInertia=Iprop_yz_zx_xy  ProductsOfInertiaUnits=kg*m^2  DensityBased=on  Density=1000  DensityUnits=kg/(m^3)  DoExposeReferenceFrame=on  SerializedFrames=<Frames/>  GraphicType=FromGeometry  MarkerShape=Sphere  MarkerSize=10  MarkerSizeUnits=m  GraphicVisPropType=SimpleVisualProperties  GraphicDiffuseColor=[1.0 1.0 0.0]  GraphicSpecularColor=[0.5 0.5 0.5 1.0]  GraphicAmbientColor=[0.15 0.15 0.15 1.0]  GraphicEmissiveColor=[0.0 0.0 0.0 1.0]  GraphicShininess=75  GraphicOpacity=1.0  GeometryShape=Cylinder  RectangleSize=[1 1]  RectangleSizeUnits=m  BrickDimensions=[1 1 1]  BrickDimensionUnits=m  CylinderRadius=prop_CG_H  CylinderRadiusUnits=m  CylinderLength=2*prop_CG_H  CylinderLengthUnits=m  SphereRadius=1  SphereRadiusUnits=m  EllipsoidRadii=[prop_CG_L, prop_CG_L, prop_CG_L/10]  EllipsoidRadiiUnits=m  ExtrusionCrossSection=[1 1; -1 1; -1 -1; 1 -1]  ExtrusionCrossSectionUnits=m  ExtrusionLength=1  ExtrusionLengthUnits=m  PolygonNumSides=3  PolygonOuterRadius=1  PolygonOuterRadiusUnits=m  ExtGeomFileType=STL  ExtGeomFileUnits=m  RevolutionCrossSection=[1 1; 1 -1; 2 -1; 2 1]  RevolutionCrossSectionUnits=m  RevolutionExtent=Full  RevolutionAngle=180  RevolutionAngleUnits=deg
      settings: AttributesFormatString=|
      | %<Mass>
      | %<MomentsOfInertia>
      | %<ProductsOfInertia>
  PROP_4 : sm_lib/Body Elements/Solid  InertiaType=Custom  Mass=prop_mass  MassUnits=kg  CenterOfMass=[0 0 0]  CenterOfMassUnits=m  MomentsOfInertia=Iprop_xx_yy_zz  MomentsOfInertiaUnits=kg*m^2  ProductsOfInertia=Iprop_yz_zx_xy  ProductsOfInertiaUnits=kg*m^2  DensityBased=on  Density=1000  DensityUnits=kg/(m^3)  DoExposeReferenceFrame=on  SerializedFrames=<Frames/>  GraphicType=FromGeometry  MarkerShape=Sphere  MarkerSize=10  MarkerSizeUnits=m  GraphicVisPropType=SimpleVisualProperties  GraphicDiffuseColor=[0.2 1.0 1.0]  GraphicSpecularColor=[0.5 0.5 0.5 1.0]  GraphicAmbientColor=[0.15 0.15 0.15 1.0]  GraphicEmissiveColor=[0.0 0.0 0.0 1.0]  GraphicShininess=75  GraphicOpacity=1.0  GeometryShape=Cylinder  RectangleSize=[1 1]  RectangleSizeUnits=m  BrickDimensions=[1 1 1]  BrickDimensionUnits=m  CylinderRadius=prop_CG_H  CylinderRadiusUnits=m  CylinderLength=2*prop_CG_H  CylinderLengthUnits=m  SphereRadius=1  SphereRadiusUnits=m  EllipsoidRadii=[prop_CG_L, prop_CG_L, prop_CG_L/10]  EllipsoidRadiiUnits=m  ExtrusionCrossSection=[1 1; -1 1; -1 -1; 1 -1]  ExtrusionCrossSectionUnits=m  ExtrusionLength=1  ExtrusionLengthUnits=m  PolygonNumSides=3  PolygonOuterRadius=1  PolygonOuterRadiusUnits=m  ExtGeomFileType=STL  ExtGeomFileUnits=m  RevolutionCrossSection=[1 1; 1 -1; 2 -1; 2 1]  RevolutionCrossSectionUnits=m  RevolutionExtent=Full  RevolutionAngle=180  RevolutionAngleUnits=deg
      settings: AttributesFormatString=|
      | %<Mass>
      | %<MomentsOfInertia>
      | %<ProductsOfInertia>
  RT_air2prop1 : sm_lib/Frames and Transforms/Rigid Transform  TranslationMethod=Cartesian  TranslationStandardOffset=0  TranslationLengthUnit=m  TranslationStandardAxis=+Z  TranslationCartesianOffset=[prop_CG_L, 0, prop_CG_H]  TranslationROffset=0  TranslationROffsetUnits=m  TranslationZOffset=0  TranslationZOffsetUnits=m  TranslationThetaOffset=0  TranslationThetaOffsetUnits=deg  RotationMethod=None  RotationAngleUnits=deg  RotationStandardAxis=+Z  RotationAngle=0  RotationArbitraryAxis=[0 0 1]  FollAlignAxisA=+X  BaseAlignAxisA=+Y  FollAlignAxisB=+Y  BaseAlignAxisB=+Z  RotationSequenceAxes=FollowerAxes  RotationSequence=XYX  RotationSequenceAngles=[0 0 0]  RotationSequenceAnglesUnits=deg  RotationMatrix=[1 0 0; 0 1 0; 0 0 1]
  RT_air2prop2 : sm_lib/Frames and Transforms/Rigid Transform  TranslationMethod=Cartesian  TranslationStandardOffset=0  TranslationLengthUnit=m  TranslationStandardAxis=+Z  TranslationCartesianOffset=[0,prop_CG_L, prop_CG_H]  TranslationROffset=0  TranslationROffsetUnits=m  TranslationZOffset=0  TranslationZOffsetUnits=m  TranslationThetaOffset=0  TranslationThetaOffsetUnits=deg  RotationMethod=None  RotationAngleUnits=deg  RotationStandardAxis=+Z  RotationAngle=0  RotationArbitraryAxis=[0 0 1]  FollAlignAxisA=+X  BaseAlignAxisA=+Y  FollAlignAxisB=+Y  BaseAlignAxisB=+Z  RotationSequenceAxes=FollowerAxes  RotationSequence=XYX  RotationSequenceAngles=[0 0 0]  RotationSequenceAnglesUnits=deg  RotationMatrix=[1 0 0; 0 1 0; 0 0 1]
  RT_air2prop3 : sm_lib/Frames and Transforms/Rigid Transform  TranslationMethod=Cartesian  TranslationStandardOffset=0  TranslationLengthUnit=m  TranslationStandardAxis=+Z  TranslationCartesianOffset=[-prop_CG_L, 0, prop_CG_H]  TranslationROffset=0  TranslationROffsetUnits=m  TranslationZOffset=0  TranslationZOffsetUnits=m  TranslationThetaOffset=0  TranslationThetaOffsetUnits=deg  RotationMethod=None  RotationAngleUnits=deg  RotationStandardAxis=+Z  RotationAngle=0  RotationArbitraryAxis=[0 0 1]  FollAlignAxisA=+X  BaseAlignAxisA=+Y  FollAlignAxisB=+Y  BaseAlignAxisB=+Z  RotationSequenceAxes=FollowerAxes  RotationSequence=XYX  RotationSequenceAngles=[0 0 0]  RotationSequenceAnglesUnits=deg  RotationMatrix=[1 0 0; 0 1 0; 0 0 1]
  RT_air2prop4 : sm_lib/Frames and Transforms/Rigid Transform  TranslationMethod=Cartesian  TranslationStandardOffset=0  TranslationLengthUnit=m  TranslationStandardAxis=+Z  TranslationCartesianOffset=[0,-prop_CG_L, prop_CG_H]  TranslationROffset=0  TranslationROffsetUnits=m  TranslationZOffset=0  TranslationZOffsetUnits=m  TranslationThetaOffset=0  TranslationThetaOffsetUnits=deg  RotationMethod=None  RotationAngleUnits=deg  RotationStandardAxis=+Z  RotationAngle=0  RotationArbitraryAxis=[0 0 1]  FollAlignAxisA=+X  BaseAlignAxisA=+Y  FollAlignAxisB=+Y  BaseAlignAxisB=+Z  RotationSequenceAxes=FollowerAxes  RotationSequence=XYX  RotationSequenceAngles=[0 0 0]  RotationSequenceAnglesUnits=deg  RotationMatrix=[1 0 0; 0 1 0; 0 0 1]
  Selector1 : Selector  InputPortWidth=4  IndexOptions=Index vector (dialog)  Indices=2  OutputSizes=1
  Selector2 : Selector  InputPortWidth=4  IndexOptions=Index vector (dialog)  Indices=3  OutputSizes=1
  Selector3 : Selector  InputPortWidth=4  IndexOptions=Index vector (dialog)  Indices=4  OutputSizes=1
  Selector4 : Selector  InputPortWidth=4  IndexOptions=Index vector (dialog)  Indices=1  OutputSizes=1
  Selector5 : Selector  InputPortWidth=4  IndexOptions=Index vector (dialog)  Indices=2  OutputSizes=1
  Selector6 : Selector  InputPortWidth=4  IndexOptions=Index vector (dialog)  Indices=3  OutputSizes=1
  Selector7 : Selector  InputPortWidth=4  IndexOptions=Index vector (dialog)  Indices=4  OutputSizes=1
  Selector8 : Selector  InputPortWidth=4  IndexOptions=Index vector (dialog)  Indices=1  OutputSizes=1
  Simulink-PS Converter{,1..3} (4 alike) : nesl_utility/Simulink-PS Converter  PhysicalDomain=network_engine_domain  SubClassName=ps_input  LeftPortType=input  RightPortType=output  PseudoPeriodic=off  Frequencies=[]  NoiseDistribution=none  NoiseParameters=[]  Unit=N*m  AffineConversion=off  FilteringAndDerivatives=provide  SimscapeFilterOrder=1  InputFilterTimeConstant=0.001  UdotUserProvided=0
  Simulink-PS Converter{4..7} (4 alike) : nesl_utility/Simulink-PS Converter  PhysicalDomain=network_engine_domain  SubClassName=ps_input  LeftPortType=input  RightPortType=output  PseudoPeriodic=off  Frequencies=[]  NoiseDistribution=none  NoiseParameters=[]  Unit=N  AffineConversion=off  FilteringAndDerivatives=provide  SimscapeFilterOrder=1  InputFilterTimeConstant=0.001  UdotUserProvided=0
  THRUST_{1..4} (4 alike) : sm_lib/Forces and Torques/External Force and Torque  ForceResolutionFrame=AttachedFrame  EnableForceX=off  EnableForceY=off  EnableForceZ=on  EnableForce=off  TorqueResolutionFrame=AttachedFrame  EnableTorqueX=off  EnableTorqueY=off  EnableTorqueZ=on  EnableTorque=off
  joint_prop{1..4} (4 alike) : sm_lib/Joints/Revolute Joint  SenseConstraintForce=off  SenseConstraintForceX=off  SenseConstraintForceY=off  SenseConstraintForceZ=off  SenseConstraintTorque=off  SenseConstraintTorqueX=off  SenseConstraintTorqueY=off  SenseConstraintTorqueZ=off  SenseTotalForce=off  SenseTotalForceX=off  SenseTotalForceY=off  SenseTotalForceZ=off  SenseTotalTorque=off  SenseTotalTorqueX=off  SenseTotalTorqueY=off  SenseTotalTorqueZ=off  CompositeWrenchDir=FollowerOnBase  CompositeWrenchFrame=BaseFrame  EquilibriumPosition=0  EquilibriumPositionUnits=deg  SpringStiffness=0  SpringStiffnessUnits=N*m/deg  DampingCoefficient=0  DampingCoefficientUnits=N*m/(deg/s)  TorqueActuationMode=NoTorque  MotionActuationMode=ComputedMotion  SensePosition=off  SenseVelocity=off  SenseAcceleration=off  SenseTorqueForce=off  PositionTargetSpecify=off  PositionTargetPriority=High  PositionTargetValue=0  PositionTargetValueUnits=deg  VelocityTargetSpecify=off  VelocityTargetPriority=High  VelocityTargetValue=0  VelocityTargetValueUnits=deg/s
  airCG : PMIOPort  Port=1  Side=Left
  wires:
  mot_TQ_vec/1 -> [TQ]
  mot_THRUST_vec/1 -> [Fb]
  Selector4/1 -> Simulink-PS Converter7/1
  [Fb] -> Selector4/1
  Selector5/1 -> Simulink-PS Converter6/1
  [Fb] -> Selector5/1
  Selector6/1 -> Simulink-PS Converter5/1
  [Fb] -> Selector6/1
  Selector7/1 -> Simulink-PS Converter4/1
  [Fb] -> Selector7/1
  mot_speed_vec/1 -> [w]
  [TQ] -> Selector8/1
  Selector8/1 -> Simulink-PS Converter/1
  [TQ] -> Selector1/1
  Selector1/1 -> Simulink-PS Converter1/1
  [TQ] -> Selector2/1
  Selector2/1 -> Simulink-PS Converter2/1
  [TQ] -> Selector3/1
  Selector3/1 -> Simulink-PS Converter3/1
  connections:
  RT_air2prop1/LConn1 -- airCG/RConn1 -- RT_air2prop2/LConn1 -- RT_air2prop3/LConn1 -- RT_air2prop4/LConn1
  PROP_1/RConn1 -- joint_prop1/RConn1
  RT_air2prop1/RConn1 -- THRUST_1/RConn1 -- joint_prop1/LConn1
  joint_prop2/LConn1 -- THRUST_2/RConn1 -- RT_air2prop2/RConn1
  joint_prop2/RConn1 -- PROP_2/RConn1
  joint_prop4/LConn1 -- THRUST_4/RConn1 -- RT_air2prop4/RConn1
  joint_prop3/LConn1 -- THRUST_3/RConn1 -- RT_air2prop3/RConn1
  joint_prop4/RConn1 -- PROP_4/RConn1
  joint_prop3/RConn1 -- PROP_3/RConn1
  Simulink-PS Converter7/RConn1 -- THRUST_1/LConn1
  Simulink-PS Converter/RConn1 -- THRUST_1/LConn2
  THRUST_2/LConn1 -- Simulink-PS Converter6/RConn1
  Simulink-PS Converter1/RConn1 -- THRUST_2/LConn2
  Simulink-PS Converter2/RConn1 -- THRUST_3/LConn2
  Simulink-PS Converter5/RConn1 -- THRUST_3/LConn1
  THRUST_4/LConn1 -- Simulink-PS Converter4/RConn1
  Simulink-PS Converter3/RConn1 -- THRUST_4/LConn2

== system bh_SM_quad_NO_spin_props/MODEL_SYS/bh_6DOF (Simscape)/echo_MASK_params ==
  Constant : Constant  Value=air_mass_0  OutDataTypeStr=Inherit: Inherit via back propagation
  Constant1 : Constant  Value=air_inertia_0  OutDataTypeStr=Inherit: Inherit via back propagation
  Constant11 : Constant  Value=xme_0  OutDataTypeStr=Inherit: Inherit via back propagation
  Constant2 : Constant  Value=prop_Imat  OutDataTypeStr=Inherit: Inherit via back propagation
  Constant3 : Constant  Value=prop_CG_L  OutDataTypeStr=Inherit: Inherit via back propagation
  Constant4 : Constant  Value=prop_CG_H  OutDataTypeStr=Inherit: Inherit via back propagation
  Constant5 : Constant  Value=prop_mass  OutDataTypeStr=Inherit: Inherit via back propagation
  Constant6 : Constant  Value=g_const  OutDataTypeStr=Inherit: Inherit via back propagation
  Constant7 : Constant  Value=eul_0  OutDataTypeStr=Inherit: Inherit via back propagation
  Constant8 : Constant  Value=Vm_0  OutDataTypeStr=Inherit: Inherit via back propagation
  Constant9 : Constant  Value=pm_0  OutDataTypeStr=Inherit: Inherit via back propagation
  Display{,1..10} (11 alike) : Display
  Reshape{1..3,5} (4 alike) : Reshape  OutputDimensionality=Column vector (2-D)
  wires:
  Constant2/1 -> Display1/1
  Constant1/1 -> Display/1
  Constant4/1 -> Display2/1
  Constant6/1 -> Display4/1
  Constant/1 -> Display5/1
  Constant5/1 -> Display6/1
  Constant3/1 -> Display3/1
  Constant7/1 -> Reshape5/1
  Reshape5/1 -> Display7/1
  Reshape1/1 -> Display8/1
  Constant9/1 -> Reshape1/1
  Reshape2/1 -> Display9/1
  Constant8/1 -> Reshape2/1
  Reshape3/1 -> Display10/1
  Constant11/1 -> Reshape3/1
